simulink model "s6_template"  (R2019a)
settings: Solver=ode4  StartTime=0.0  StopTime=inf  FixedStep=P_sim_dt  RelTol=1e-3
InitFcn:
  | s6_data;
values from neighbouring files (symbols this model uses):
  CarInputsCmdForward = uint8(1)    [p_mad_car.m]
libraries: mad_lib_template x1
settings Model: EnablePacing=on  Creator=hmekiedj  LastModifiedBy=frank
settings DataIOCC: ReturnWorkspaceOutputs=off
settings DebuggingCC: ArithmeticOperatorsInVariantConditions=warning
settings SFSimCC: SimUseLocalCustomCode=off
settings RTWCC: RTWUseLocalCustomCode=off
settings CodeAppCC: StateflowObjectComments=on

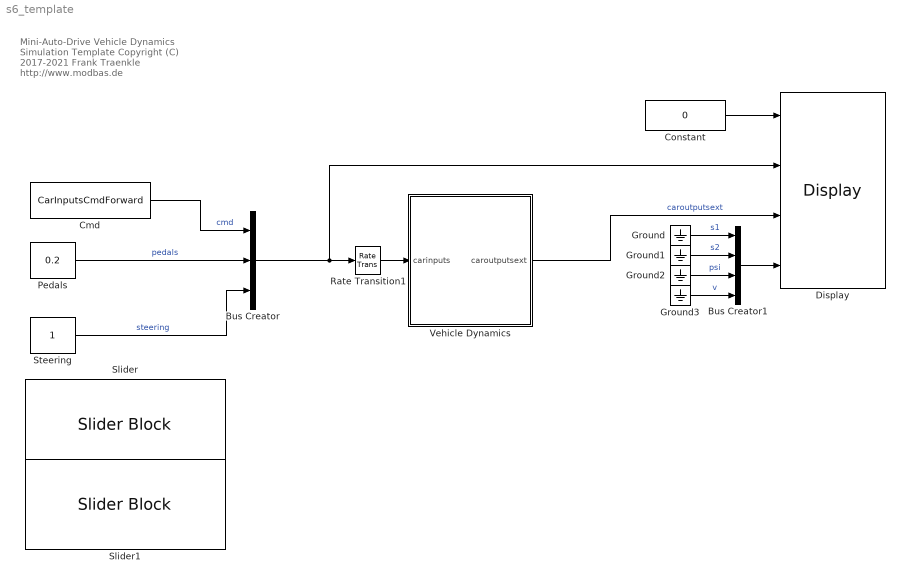
== system s6_template ==
  note: Mini-Auto-Drive
      | Vehicle Dynamics Simulation Template
      | Copyright (C) 2017-2021 Frank Traenkle
      | http://www.modbas.de
  Bus Creator : BusCreator  Inputs=3
  Bus Creator1 : BusCreator  Inputs=4
  Cmd : Constant  Value=CarInputsCmdForward  SampleTime=-1
  Constant : Constant  Value=0
  Display : mad_lib_template/Display  SystemSampleTime=-1
  Ground{,1..3} (4 alike) : Ground
  Pedals : Constant  Value=0.2  SampleTime=-1
  Rate Transition1 : RateTransition
  Slider : SliderBlock  ScaleMin=-1  ScaleMax=1
  Slider1 : SliderBlock  LabelPosition=Bottom  ScaleMin=-1  ScaleMax=1
  Steering : Constant  SampleTime=-1
  Vehicle Dynamics : Subsystem
  wires:
  Pedals/1 -> Bus Creator/2  "pedals"
  Bus Creator1/1 -> Display/4
  Ground/1 -> Bus Creator1/1  "s1"
  Ground1/1 -> Bus Creator1/2  "s2"
  Ground2/1 -> Bus Creator1/3  "psi"
  Ground3/1 -> Bus Creator1/4  "v"
  Vehicle Dynamics/1(caroutputsext) -> Display/3  "caroutputsext"
  Steering/1 -> Bus Creator/3  "steering"
  Bus Creator/1 -> Display/2, Rate Transition1/1
  Rate Transition1/1 -> Vehicle Dynamics/1(carinputs)
  Constant/1 -> Display/1
  Cmd/1 -> Bus Creator/1  "cmd"

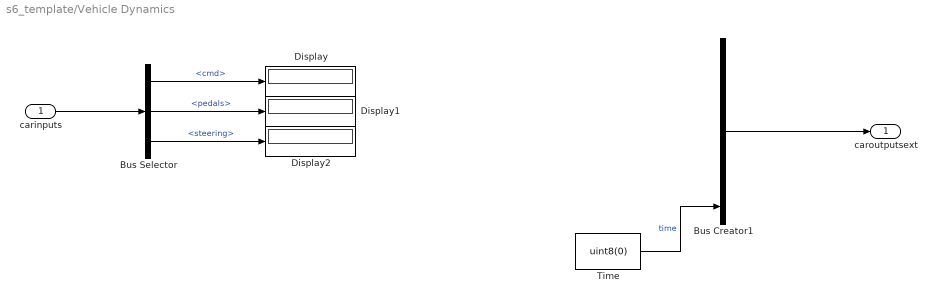
== system s6_template/Vehicle Dynamics ==
  carinputs : Inport
  Bus Creator1 : BusCreator  Inputs=7  OutDataTypeStr=Bus: CAROUTPUTSEXT
  Bus Selector : BusSelector  OutputSignals=cmd,pedals,steering
  Display : Display
  Display1 : Display
  Display2 : Display
  Time : Constant  Value=uint8(0)
  caroutputsext : Outport
  wires:
  carinputs/1 -> Bus Selector/1
  Bus Selector/2 -> Display1/1  "<pedals>"
  Bus Selector/3 -> Display2/1  "<steering>"
  ? -> Bus Creator1/3  "psi"
  ? -> Bus Creator1/5  "v"
  Bus Creator1/1 -> caroutputsext/1
  ? -> Bus Creator1/6  "x"
  ? -> Bus Creator1/2  "s2"
  ? -> Bus Creator1/4  "beta"
  ? -> Bus Creator1/1  "s1"
  Time/1 -> Bus Creator1/7  "time"
  Bus Selector/1 -> Display/1  "<cmd>"
